simulink model "test"  (R2020b)
settings: Solver=VariableStepAuto  StartTime=0.0  StopTime=10.0  RelTol=1e-3
undefined symbols (not defined in the file or in its folder): A_kalman, L
libraries: simulink x1
settings Model: Creator=renato  LastModifiedBy=renato

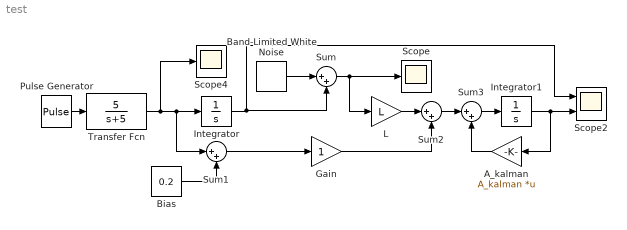
== system test ==
  A_kalman : Gain  Gain=A_kalman  Multiplication=Matrix(K*u)
  Band-Limited White Noise : simulink/Sources/Band-Limited White Noise  Cov=[0.000001]  Ts=0.1  seed=[23341]
  Bias : Constant  Value=0.2
  Gain : Gain
  Integrator : Integrator
  Integrator1 : Integrator
  L : Gain  Gain=L
  Pulse Generator : DiscretePulseGenerator  PulseType=Time based  Amplitude=0.1  Period=10  PulseWidth=10  PhaseDelay=1
  Scope : Scope
  Scope2 : Scope  NumInputPorts=2
  Scope4 : Scope
  Sum{,1..3} (4 alike) : Sum  Inputs=|++
  Transfer Fcn : TransferFcn  Numerator=[5]  Denominator=[1 5]
  wires:
  Integrator/1 -> Sum/2, Scope2/1
  Pulse Generator/1 -> Transfer Fcn/1
  Sum/1 -> L/1, Scope/1
  Sum1/1 -> Gain/1
  L/1 -> Sum2/1
  A_kalman/1 -> Sum3/2
  Sum2/1 -> Sum3/1
  Sum3/1 -> Integrator1/1
  Gain/1 -> Sum2/2
  Band-Limited White Noise/1 -> Sum/1
  Integrator1/1 -> Scope2/2, A_kalman/1
  Transfer Fcn/1 -> Scope4/1, Sum1/1, Integrator/1
  Bias/1 -> Sum1/2
